simulink model "ball1"  (Simulink 2.00)
settings: Solver=ode45  StartTime=0.0  StopTime=10.0  RelTol=1e-3  AbsTol=1e-6
undefined symbols (not defined in the file or in its folder): sfunxy
settings Model: ConsistencyChecking=off

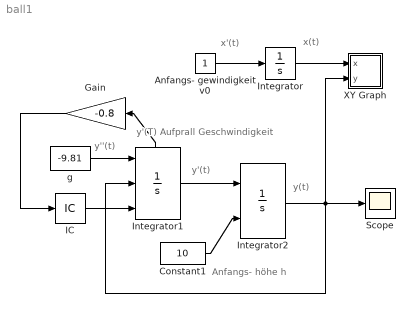
== system ball1 ==
  note: x'(t)
  note: x(t)
  note: Anfangs-
      | höhe h
  note: y''(t)
  note: y'(t)
  note: y(t)
  note: y'(T) Aufprall
      | Geschwindigkeit
  Anfangs- gewindigkeit v0 : Constant  Value=1
  Constant1 : Constant  Value=10
  Gain : Gain  Orientation=left  Gain=-0.8
  IC : InitialCondition  Value=0
  Integrator : Integrator  ExternalReset=none  InitialConditionSource=internal  InitialCondition=0  LimitOutput=off  UpperSaturationLimit=inf  LowerSaturationLimit=-inf  ShowSaturationPort=off  ShowStatePort=off  AbsoluteTolerance=auto
  Integrator1 : Integrator  ExternalReset=falling  InitialConditionSource=external  InitialCondition=0  LimitOutput=off  UpperSaturationLimit=inf  LowerSaturationLimit=-inf  ShowSaturationPort=off  ShowStatePort=on  AbsoluteTolerance=auto
  Integrator2 : Integrator  ExternalReset=none  InitialConditionSource=external  InitialCondition=0  LimitOutput=on  UpperSaturationLimit=inf  LowerSaturationLimit=0  ShowSaturationPort=off  ShowStatePort=off  AbsoluteTolerance=auto
  Scope : Scope
      settings: TickLabels=on  TimeRange=10  YMin=0  YMax=10  SaveToWorkspace=off  SaveName=ScopeData
  XY Graph : Subsystem  mask(XY scope.){ax(1)=0, ax(2)=10, ax(3)=0, ax(4)=10, st=-1}
      mask prompts: ax(1) "x-min"; ax(2) "x-max"; ax(3) "y-min"; ax(4) "y-max"; st "Sample Time"
      mask help: XY scope using MATLAB graph window. First input is used as time base. Enter plotting ranges.
      mask Help: This block can be used to explore limit cycles. Look at the m-file sfunxy.m to see how it works.
      mask Display: plot([.05 .95 .95 .05 .05],[.45 .45 .95 .95 .45], 0.5+cos(0:0.1:2*pi)*0.3,0.7+sin(0:0.1:2*pi)*0.2)
  g : Constant  Value=-9.81
  wires:
  Integrator1/1 -> Integrator2/1
  Constant1/1 -> Integrator2/2
  IC/1 -> Integrator1/3
  Integrator1/State -> Gain/1
  Gain/1 -> IC/1
  g/1 -> Integrator1/1
  Integrator2/1 -> Integrator1/2, Scope/1, XY Graph/2(y)
  Anfangs- gewindigkeit v0/1 -> Integrator/1
  Integrator/1 -> XY Graph/1(x)

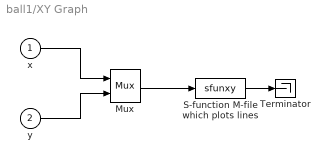
== system ball1/XY Graph ==
  x : Inport  Port=1  PortWidth=-1  SampleTime=-1
  y : Inport  Port=2  PortWidth=-1  SampleTime=-1
  Mux : Mux  Inputs=2
  "S-function M-file which plots lines " : S-Function  LoadFcn=sfunxy([],[],[],'LoadBlock')  FunctionName=sfunxy  Parameters=ax, st
      settings: CopyFcn=sfunxy([],[],[],'CopyBlock')  DeleteFcn=sfunxy([],[],[],'DeleteBlock')
  Terminator : Terminator
  wires:
  "S-function M-file which plots lines "/1 -> Terminator/1
  y/1 -> Mux/2
  x/1 -> Mux/1
  Mux/1 -> "S-function M-file which plots lines "/1
